simulink model "Binarisation_final_19821"  (R2018b)
settings: Solver=VariableStepAuto  StartTime=0.0  StopTime=10.0  RelTol=1e-3
libraries: visionsources x1, dspmtrx3 x1
settings Model: Creator=Administrator  LastModifiedBy=Administrator
settings OptimizationCC: BlockReduction=off  ConditionallyExecuteInputs=off  DefaultParameterBehavior=Inlined
settings DebuggingCC: AlgebraicLoopMsg=error
settings HardwareCC: ProdBitPerPointer=32  ProdBitPerSizeT=32  ProdBitPerPtrDiffT=32  ProdLargestAtomicFloat=None  ProdIntDivRoundTo=Undefined  ProdEndianess=Unspecified  ProdWordSize=32  ProdHWDeviceType=ASIC/FPGA->ASIC/FPGA  TargetBitPerPointer=64  TargetBitPerSizeT=64  TargetBitPerPtrDiffT=64  TargetLongLongMode=on  TargetIntDivRoundTo=Zero  TargetEndianess=LittleEndian  TargetWordSize=64  TargetHWDeviceType=Custom Processor->MATLAB Host Computer  ProdEqTarget=off

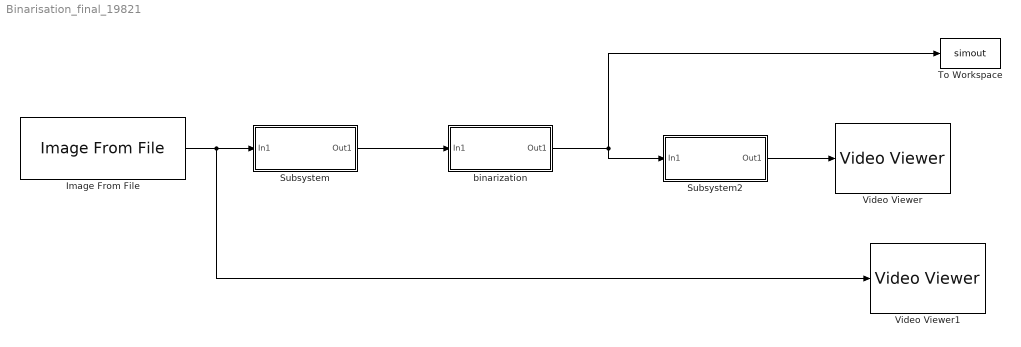
== system Binarisation_final_19821 ==
  Image From File : visionsources/Image From File  Tag=vipblks_nd  FileName=C:\Users\Administrator\Desktop\Meeting_23.1.2021\segmentation\16821\output.bmp  imagePorts=One multidimensional signal  Ts=0.1  ImageDataType=uint8  Signed=on  WordLength=16  sdImageDataType=uint(8)  FractionLengthMode=User-defined  FractionLength=15  OutPortLabels=R|G|B
      settings: SourceProductName=Computer Vision System Toolbox
  Subsystem : Subsystem
  Subsystem2 : Subsystem
  To Workspace : ToWorkspace  VariableName=simout  SampleTime=-1
  Video Viewer : VideoViewer  FigPos=[1042 1066 418 461]
  Video Viewer1 : VideoViewer  FigPos=[184 1000 418 304]
  binarization : Subsystem  TreatAsAtomicUnit=on
  wires:
  Subsystem2/1(Out1) -> Video Viewer/1
  Image From File/1 -> Video Viewer1/1, Subsystem/1(In1)
  Subsystem/1(Out1) -> binarization/1(In1)
  binarization/1(Out1) -> Subsystem2/1(In1), To Workspace/1

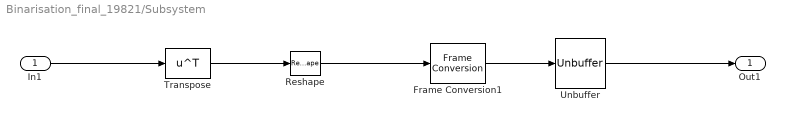
== system Binarisation_final_19821/Subsystem ==
  In1 : Inport
  Frame Conversion1 : FrameConversion
  Reshape : Reshape
  Transpose : Math  Operator=transpose  RndMeth=Zero  SaturateOnIntegerOverflow=on
  Unbuffer : Unbuffer  ic=1
  Out1 : Outport
  wires:
  Reshape/1 -> Frame Conversion1/1
  In1/1 -> Transpose/1
  Frame Conversion1/1 -> Unbuffer/1
  Unbuffer/1 -> Out1/1
  Transpose/1 -> Reshape/1

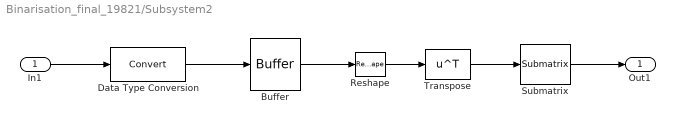
== system Binarisation_final_19821/Subsystem2 ==
  In1 : Inport
  Buffer : Buffer  N=65536  OutputFrames=off
  Data Type Conversion : DataTypeConversion
  Reshape : Reshape  OutputDimensionality=Customize  OutputDimensions=[256,256]
  Submatrix : dspmtrx3/Submatrix  RowSpan=Range of rows  RowStartMode=First  RowStartIndex=1  RowEndMode=Last  RowEndIndex=1  ColSpan=Range of columns  ColStartMode=First  ColStartIndex=1  ColEndMode=Last  ColEndIndex=1
  Transpose : Math  Operator=transpose  RndMeth=Zero  SaturateOnIntegerOverflow=on
  Out1 : Outport
  wires:
  Data Type Conversion/1 -> Buffer/1
  Buffer/1 -> Reshape/1
  Reshape/1 -> Transpose/1
  Transpose/1 -> Submatrix/1
  Submatrix/1 -> Out1/1
  In1/1 -> Data Type Conversion/1

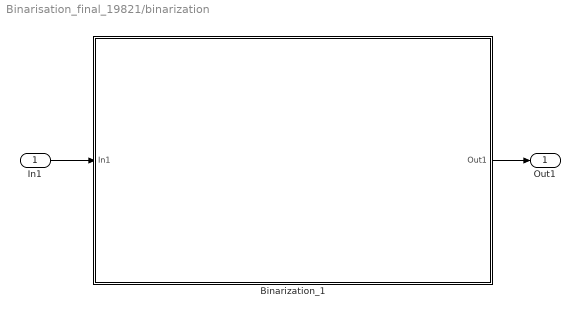
== system Binarisation_final_19821/binarization ==
  In1 : Inport
  Binarization_1 : Subsystem  TreatAsAtomicUnit=on
  Out1 : Outport
  wires:
  In1/1 -> Binarization_1/1(In1)
  Binarization_1/1(Out1) -> Out1/1

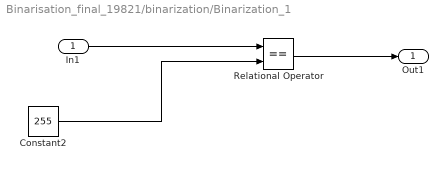
== system Binarisation_final_19821/binarization/Binarization_1 ==
  In1 : Inport
  Constant2 : Constant  Value=255  OutDataTypeStr=fixdt(1,16)  SampleTime=-1
  Relational Operator : RelationalOperator  Operator===  OutDataTypeStr=boolean  RndMeth=Nearest
  Out1 : Outport
  wires:
  Constant2/1 -> Relational Operator/2
  In1/1 -> Relational Operator/1
  Relational Operator/1 -> Out1/1
